simulink model "simu_red_adelanto"  (R2020b)
settings: Solver=VariableStepAuto  StartTime=0.0  StopTime=6  RelTol=1e-3
values from neighbouring files (symbols this model uses):
  K = 4    [adelanto_ao.m]    (also in compensador_adelanto.m = 1/div)
  p = 4    [adelanto_ao.m]    (also in compensador_adelanto.m = 6.13120784795)
  z = 2    [adelanto_ao.m]    (also in compensador_adelanto.m = 8)
settings Model: Creator=cmparedes  LastModifiedBy=Acer

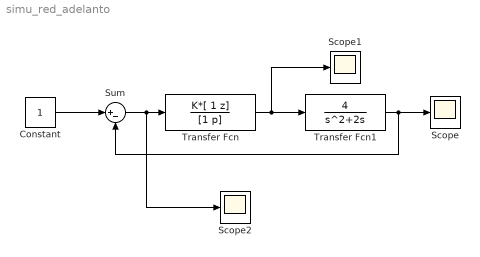
== system simu_red_adelanto ==
  Constant : Constant
  Scope : Scope
  Scope1 : Scope
  Scope2 : Scope
  Sum : Sum  Inputs=|+-
  Transfer Fcn : TransferFcn  Numerator=K*[ 1 z]  Denominator=[1 p]
  Transfer Fcn1 : TransferFcn  Numerator=[4]  Denominator=[1 2 0]
  wires:
  Sum/1 -> Scope2/1, Transfer Fcn/1
  Transfer Fcn/1 -> Scope1/1, Transfer Fcn1/1
  Transfer Fcn1/1 -> Sum/2, Scope/1
  Constant/1 -> Sum/1
